simulink model "DC_Motor_Cascade_vs_Single_PI"  (R2021a)
settings: Solver=FixedStepAuto  StartTime=0.0  StopTime=3  FixedStep=1e-4  RelTol=1e-3
values from neighbouring files (symbols this model uses):
  B = 0.002    [motor_params.m]
  J = 0.05    [motor_params.m]
  Ke = 1.5    [motor_params.m]
  Kt = 1.5    [motor_params.m]
  L = 0.02    [motor_params.m]
  R = 2.5    [motor_params.m]
  V_nom = 240    [motor_params.m]
libraries: pid_lib x3, simulink x2
settings Model: SimulationMode=accelerator  Creator=DELL  LastModifiedBy=DELL

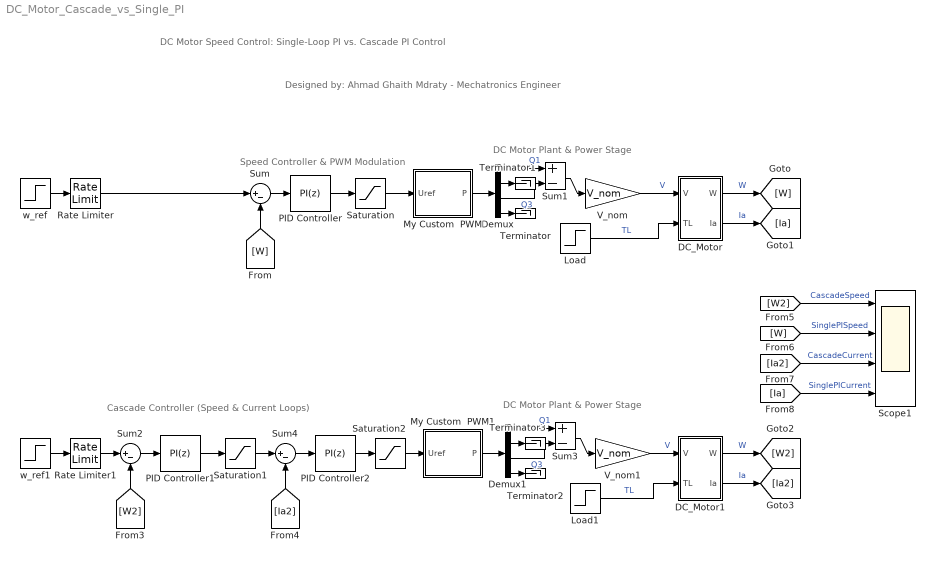
== system DC_Motor_Cascade_vs_Single_PI ==
  note: DC Motor Speed Control: Single-Loop PI vs. Cascade PI Control
  note: DC Motor Plant & Power Stage
  note: Cascade Controller (Speed & Current Loops)
  note: DC Motor Plant & Power Stage
  note: Speed Controller & PWM Modulation
  note: Designed by: Ahmad Ghaith Mdraty - Mechatronics Engineer
  DC_Motor : Subsystem
  DC_Motor1 : Subsystem
  Demux : Demux
  Demux1 : Demux
  Load : Step  Time=2  Before=1  After=20  SampleTime=0
  Load1 : Step  Time=2  Before=1  After=20  SampleTime=0
  My Custom  PWM : Subsystem  mask{PWM_Mode=Unipolar}
      mask prompts: PWM_Mode "Select PWM Modulation:"
      mask TypeOptions PWM_Mode: Bipolar | Unipolar
  My Custom  PWM1 : Subsystem  mask{PWM_Mode=Unipolar}
      mask prompts: PWM_Mode "Select PWM Modulation:"
      mask TypeOptions PWM_Mode: Bipolar | Unipolar
  PID Controller : pid_lib/PID Controller  Controller=PI  Form=Parallel  TimeDomain=Discrete-time  UseExternalTs=off  SampleTime=-1  IntegratorMethod=Forward Euler  FilterMethod=Forward Euler  ControllerParametersSource=internal  P=0.05  I=2  D=0  UseFilter=on  N=100  TunerSelectOption=Transfer Function Based (PID Tuner App)  InitialConditionSource=internal  InitialConditionForIntegrator=0  InitialConditionForFilter=0  DifferentiatorICPrevScaledInput=0  ExternalReset=none  TrackingMode=off  Kt=1  LimitOutput=off  SatLimitsSource=internal  UpperSaturationLimit=inf  LowerSaturationLimit=-inf  LinearizeAsGain=on  AntiWindupMode=none  Kb=1  POutMin=[]  POutMax=[]  IOutMin=[]  IOutMax=[]  DOutMin=[]  DOutMax=[]  NOutMin=[]  NOutMax=[]  SumOutMin=[]  SumOutMax=[]  SaturationOutMin=[]  SaturationOutMax=[]  PParamMin=[]  PParamMax=[]  IParamMin=[]  IParamMax=[]  DParamMin=[]  DParamMax=[]  NParamMin=[]  NParamMax=[]  KbParamMin=[]  KbParamMax=[]  KtParamMin=[]  KtParamMax=[]  KbOutMin=[]  KbOutMax=[]  KtOutMin=[]  KtOutMax=[]  IntegratorOutMin=[]  IntegratorOutMax=[]  FilterOutMin=[]  FilterOutMax=[]  SumI1OutMin=[]  SumI1OutMax=[]  SumI2OutMin=[]  SumI2OutMax=[]  SumI3OutMin=[]  SumI3OutMax=[]  SumI4OutMin=[]  SumI4OutMax=[]  SumDOutMin=[]  SumDOutMax=[]  DifferentiatorOutMin=[]  DifferentiatorOutMax=[]  FilterDiffOutCoefMin=[]  FilterDiffOutCoefMax=[]  ReciprocalOutMin=[]  ReciprocalOutMax=[]  SumDenOutMin=[]  SumDenOutMax=[]  SumNumOutMin=[]  SumNumOutMax=[]  DivideOutMin=[]  DivideOutMax=[]  UdiffTsProdOutMin=[]  UdiffTsProdOutMax=[]  NTsProdOutMin=[]  NTsProdOutMax=[]  UintegralTsProdOutMin=[]  UintegralTsProdOutMax=[]  UngainTsProdOutMin=[]  UngainTsProdOutMax=[]  IntegratorContinuousStateAttributes=''  IntegratorStateMustResolveToSignalObject=off  IntegratorRTWStateStorageClass=Auto  FilterContinuousStateAttributes=''  FilterStateMustResolveToSignalObject=off  FilterRTWStateStorageClass=Auto  ParallelPVariant=InternalParameters  IdealPVariant=Disabled  IVariant=InternalParameters  DVariant=Disabled  IntegratorVariant=Discrete  SatVariant=Disabled  AWVariant=Passthrough  PCopyVariant=Disabled  TRVariant=Disabled  FdbkBlocksVariant=Forward  IdealPFdbkVariant=Disabled  SatFdbkVariant=Disabled  DerivativeFilterVariant=Disabled  NVariant=Disabled  NCopyVariant=Disabled_SignalSpec  FilterICVariant=Disabled  IntegratorICVariant=InternalICs  ExternalResetVariant=Disabled  TRSumVariant=Passthrough  SumFdbkVariant=Disabled  SumVariant=Sum_PI  TsampFilterVariant=InternalTs  TsampNgainVariant=Passthrough  TsampIntegralVariant=Passthrough  ExternalSaturationOutDataTypeStr=Inherit: Same as second input
  PID Controller1 : pid_lib/PID Controller  Controller=PI  Form=Parallel  TimeDomain=Discrete-time  UseExternalTs=off  SampleTime=-1  IntegratorMethod=Forward Euler  FilterMethod=Forward Euler  ControllerParametersSource=internal  P=8  I=40  D=0  UseFilter=on  N=100  TunerSelectOption=Transfer Function Based (PID Tuner App)  InitialConditionSource=internal  InitialConditionForIntegrator=0  InitialConditionForFilter=0  DifferentiatorICPrevScaledInput=0  ExternalReset=none  TrackingMode=off  Kt=1  LimitOutput=off  SatLimitsSource=internal  UpperSaturationLimit=inf  LowerSaturationLimit=-inf  LinearizeAsGain=on  AntiWindupMode=none  Kb=1  POutMin=[]  POutMax=[]  IOutMin=[]  IOutMax=[]  DOutMin=[]  DOutMax=[]  NOutMin=[]  NOutMax=[]  SumOutMin=[]  SumOutMax=[]  SaturationOutMin=[]  SaturationOutMax=[]  PParamMin=[]  PParamMax=[]  IParamMin=[]  IParamMax=[]  DParamMin=[]  DParamMax=[]  NParamMin=[]  NParamMax=[]  KbParamMin=[]  KbParamMax=[]  KtParamMin=[]  KtParamMax=[]  KbOutMin=[]  KbOutMax=[]  KtOutMin=[]  KtOutMax=[]  IntegratorOutMin=[]  IntegratorOutMax=[]  FilterOutMin=[]  FilterOutMax=[]  SumI1OutMin=[]  SumI1OutMax=[]  SumI2OutMin=[]  SumI2OutMax=[]  SumI3OutMin=[]  SumI3OutMax=[]  SumI4OutMin=[]  SumI4OutMax=[]  SumDOutMin=[]  SumDOutMax=[]  DifferentiatorOutMin=[]  DifferentiatorOutMax=[]  FilterDiffOutCoefMin=[]  FilterDiffOutCoefMax=[]  ReciprocalOutMin=[]  ReciprocalOutMax=[]  SumDenOutMin=[]  SumDenOutMax=[]  SumNumOutMin=[]  SumNumOutMax=[]  DivideOutMin=[]  DivideOutMax=[]  UdiffTsProdOutMin=[]  UdiffTsProdOutMax=[]  NTsProdOutMin=[]  NTsProdOutMax=[]  UintegralTsProdOutMin=[]  UintegralTsProdOutMax=[]  UngainTsProdOutMin=[]  UngainTsProdOutMax=[]  IntegratorContinuousStateAttributes=''  IntegratorStateMustResolveToSignalObject=off  IntegratorRTWStateStorageClass=Auto  FilterContinuousStateAttributes=''  FilterStateMustResolveToSignalObject=off  FilterRTWStateStorageClass=Auto  ParallelPVariant=InternalParameters  IdealPVariant=Disabled  IVariant=InternalParameters  DVariant=Disabled  IntegratorVariant=Discrete  SatVariant=Disabled  AWVariant=Passthrough  PCopyVariant=Disabled  TRVariant=Disabled  FdbkBlocksVariant=Forward  IdealPFdbkVariant=Disabled  SatFdbkVariant=Disabled  DerivativeFilterVariant=Disabled  NVariant=Disabled  NCopyVariant=Disabled_SignalSpec  FilterICVariant=Disabled  IntegratorICVariant=InternalICs  ExternalResetVariant=Disabled  TRSumVariant=Passthrough  SumFdbkVariant=Disabled  SumVariant=Sum_PI  TsampFilterVariant=InternalTs  TsampNgainVariant=Passthrough  TsampIntegralVariant=Passthrough  ExternalSaturationOutDataTypeStr=Inherit: Same as second input
  PID Controller2 : pid_lib/PID Controller  Controller=PI  Form=Parallel  TimeDomain=Discrete-time  UseExternalTs=off  SampleTime=-1  IntegratorMethod=Forward Euler  FilterMethod=Forward Euler  ControllerParametersSource=internal  P=0.1  I=15  D=0  UseFilter=on  N=100  TunerSelectOption=Transfer Function Based (PID Tuner App)  InitialConditionSource=internal  InitialConditionForIntegrator=0  InitialConditionForFilter=0  DifferentiatorICPrevScaledInput=0  ExternalReset=none  TrackingMode=off  Kt=1  LimitOutput=off  SatLimitsSource=internal  UpperSaturationLimit=inf  LowerSaturationLimit=-inf  LinearizeAsGain=on  AntiWindupMode=none  Kb=1  POutMin=[]  POutMax=[]  IOutMin=[]  IOutMax=[]  DOutMin=[]  DOutMax=[]  NOutMin=[]  NOutMax=[]  SumOutMin=[]  SumOutMax=[]  SaturationOutMin=[]  SaturationOutMax=[]  PParamMin=[]  PParamMax=[]  IParamMin=[]  IParamMax=[]  DParamMin=[]  DParamMax=[]  NParamMin=[]  NParamMax=[]  KbParamMin=[]  KbParamMax=[]  KtParamMin=[]  KtParamMax=[]  KbOutMin=[]  KbOutMax=[]  KtOutMin=[]  KtOutMax=[]  IntegratorOutMin=[]  IntegratorOutMax=[]  FilterOutMin=[]  FilterOutMax=[]  SumI1OutMin=[]  SumI1OutMax=[]  SumI2OutMin=[]  SumI2OutMax=[]  SumI3OutMin=[]  SumI3OutMax=[]  SumI4OutMin=[]  SumI4OutMax=[]  SumDOutMin=[]  SumDOutMax=[]  DifferentiatorOutMin=[]  DifferentiatorOutMax=[]  FilterDiffOutCoefMin=[]  FilterDiffOutCoefMax=[]  ReciprocalOutMin=[]  ReciprocalOutMax=[]  SumDenOutMin=[]  SumDenOutMax=[]  SumNumOutMin=[]  SumNumOutMax=[]  DivideOutMin=[]  DivideOutMax=[]  UdiffTsProdOutMin=[]  UdiffTsProdOutMax=[]  NTsProdOutMin=[]  NTsProdOutMax=[]  UintegralTsProdOutMin=[]  UintegralTsProdOutMax=[]  UngainTsProdOutMin=[]  UngainTsProdOutMax=[]  IntegratorContinuousStateAttributes=''  IntegratorStateMustResolveToSignalObject=off  IntegratorRTWStateStorageClass=Auto  FilterContinuousStateAttributes=''  FilterStateMustResolveToSignalObject=off  FilterRTWStateStorageClass=Auto  ParallelPVariant=InternalParameters  IdealPVariant=Disabled  IVariant=InternalParameters  DVariant=Disabled  IntegratorVariant=Discrete  SatVariant=Disabled  AWVariant=Passthrough  PCopyVariant=Disabled  TRVariant=Disabled  FdbkBlocksVariant=Forward  IdealPFdbkVariant=Disabled  SatFdbkVariant=Disabled  DerivativeFilterVariant=Disabled  NVariant=Disabled  NCopyVariant=Disabled_SignalSpec  FilterICVariant=Disabled  IntegratorICVariant=InternalICs  ExternalResetVariant=Disabled  TRSumVariant=Passthrough  SumFdbkVariant=Disabled  SumVariant=Sum_PI  TsampFilterVariant=InternalTs  TsampNgainVariant=Passthrough  TsampIntegralVariant=Passthrough  ExternalSaturationOutDataTypeStr=Inherit: Same as second input
  Rate Limiter : RateLimiter  RisingSlewLimit=50  FallingSlewLimit=-50  SampleTimeMode=inherited
  Rate Limiter1 : RateLimiter  RisingSlewLimit=50  FallingSlewLimit=-50  SampleTimeMode=inherited
  Saturation : Saturate  UpperLimit=1  LowerLimit=-1
  Saturation1 : Saturate  UpperLimit=15  LowerLimit=-15
  Saturation2 : Saturate  UpperLimit=1  LowerLimit=-1
  Scope1 : Scope  NumInputPorts=4
  Sum : Sum  Inputs=|+-
  Sum1 : Sum  Inputs=+-  OutDataTypeStr=double
  Sum2 : Sum  Inputs=|+-
  Sum3 : Sum  Inputs=+-  OutDataTypeStr=double
  Sum4 : Sum  Inputs=|+-
  Terminator{,1..3} (4 alike) : Terminator
  V_nom : Gain  Gain=V_nom
  V_nom1 : Gain  Gain=V_nom
  w_ref : Step  Time=0.5  After=50  SampleTime=0
  w_ref1 : Step  Time=0.5  After=50  SampleTime=0
  wires:
  DC_Motor/1(W) -> [W]  "W"
  DC_Motor/2(Ia) -> [Ia]  "Ia"
  [W] -> Sum/2
  V_nom/1 -> DC_Motor/1(V)  "V"
  Load/1 -> DC_Motor/2(TL)  "TL"
  Sum/1 -> PID Controller/1
  Saturation/1 -> My Custom  PWM/1(Uref)
  Demux/2 -> Terminator1/1
  Demux/3 -> Sum1/2  "Q3"
  PID Controller/1 -> Saturation/1
  My Custom  PWM/1(P) -> Demux/1
  w_ref/1 -> Rate Limiter/1
  Rate Limiter/1 -> Sum/1
  Demux/4 -> Terminator/1
  Demux/1 -> Sum1/1  "Q1"
  Sum1/1 -> V_nom/1
  Demux1/4 -> Terminator2/1
  Rate Limiter1/1 -> Sum2/1
  My Custom  PWM1/1(P) -> Demux1/1
  w_ref1/1 -> Rate Limiter1/1
  Demux1/2 -> Terminator3/1
  PID Controller1/1 -> Saturation1/1
  Demux1/3 -> Sum3/2  "Q3"
  DC_Motor1/1(W) -> [W2]  "W"
  Sum2/1 -> PID Controller1/1
  Sum3/1 -> V_nom1/1
  DC_Motor1/2(Ia) -> [Ia2]  "Ia"
  Load1/1 -> DC_Motor1/2(TL)  "TL"
  V_nom1/1 -> DC_Motor1/1(V)  "V"
  [W2] -> Sum2/2
  Demux1/1 -> Sum3/1  "Q1"
  Saturation1/1 -> Sum4/1
  [Ia2] -> Sum4/2
  Sum4/1 -> PID Controller2/1
  PID Controller2/1 -> Saturation2/1
  Saturation2/1 -> My Custom  PWM1/1(Uref)
  [W2] -> Scope1/1  "CascadeSpeed"
  [W] -> Scope1/2  "SinglePISpeed"
  [Ia2] -> Scope1/3  "CascadeCurrent"
  [Ia] -> Scope1/4  "SinglePICurrent"

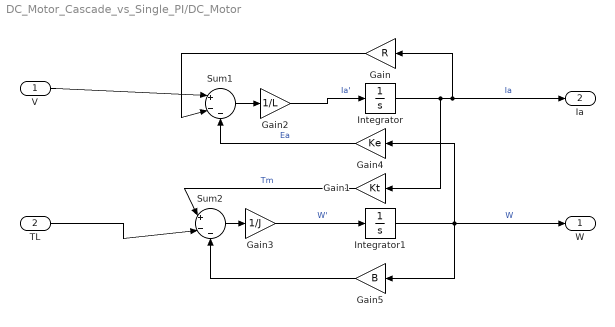
== system DC_Motor_Cascade_vs_Single_PI/DC_Motor ==
  V : Inport
  TL : Inport  Port=2
  Gain : Gain  Gain=R
  Gain1 : Gain  Gain=Kt
  Gain2 : Gain  Gain=1/L
  Gain3 : Gain  Gain=1/J
  Gain4 : Gain  Gain=Ke
  Gain5 : Gain  Gain=B
  Integrator : Integrator
  Integrator1 : Integrator
  Sum1 : Sum  Inputs=|+--
  Sum2 : Sum  Inputs=|+--
  W : Outport
  Ia : Outport  Port=2
  wires:
  TL/1 -> Sum2/2
  Integrator1/1 -> W/1, Gain5/1, Gain4/1  "W"
  Sum1/1 -> Gain2/1
  Gain/1 -> Sum1/2
  V/1 -> Sum1/1
  Gain5/1 -> Sum2/3
  Gain1/1 -> Sum2/1  "Tm"
  Gain4/1 -> Sum1/3  "Ea"
  Sum2/1 -> Gain3/1
  Integrator/1 -> Gain1/1, Ia/1, Gain/1  "Ia"
  Gain3/1 -> Integrator1/1  "W'"
  Gain2/1 -> Integrator/1  "Ia'"

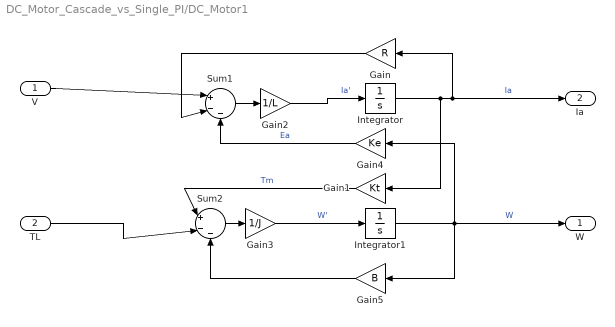
== system DC_Motor_Cascade_vs_Single_PI/DC_Motor1 ==
  V : Inport
  TL : Inport  Port=2
  Gain : Gain  Gain=R
  Gain1 : Gain  Gain=Kt
  Gain2 : Gain  Gain=1/L
  Gain3 : Gain  Gain=1/J
  Gain4 : Gain  Gain=Ke
  Gain5 : Gain  Gain=B
  Integrator : Integrator
  Integrator1 : Integrator
  Sum1 : Sum  Inputs=|+--
  Sum2 : Sum  Inputs=|+--
  W : Outport
  Ia : Outport  Port=2
  wires:
  TL/1 -> Sum2/2
  Integrator1/1 -> W/1, Gain5/1, Gain4/1  "W"
  Sum1/1 -> Gain2/1
  Gain/1 -> Sum1/2
  V/1 -> Sum1/1
  Gain5/1 -> Sum2/3
  Gain1/1 -> Sum2/1  "Tm"
  Gain4/1 -> Sum1/3  "Ea"
  Sum2/1 -> Gain3/1
  Integrator/1 -> Gain1/1, Ia/1, Gain/1  "Ia"
  Gain3/1 -> Integrator1/1  "W'"
  Gain2/1 -> Integrator/1  "Ia'"

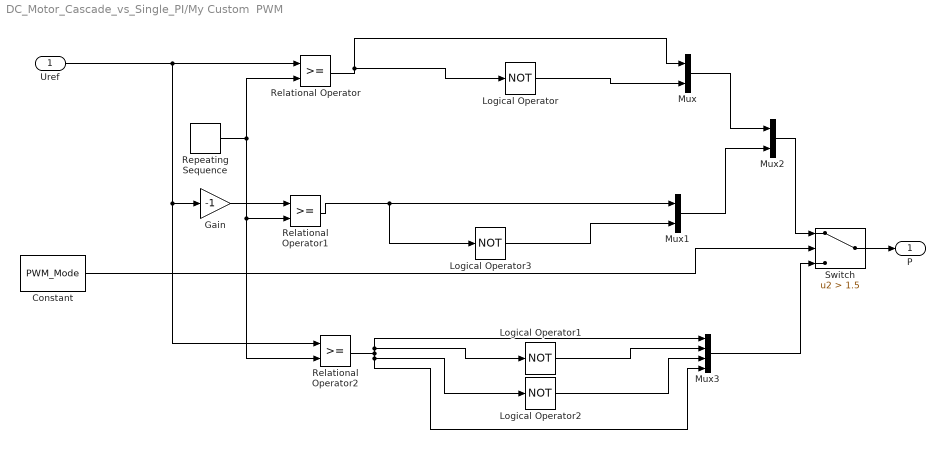
== system DC_Motor_Cascade_vs_Single_PI/My Custom  PWM ==
  Uref : Inport
  Constant : Constant  Value=PWM_Mode
  Gain : Gain  Gain=-1
  Logical Operator{,1..3} (4 alike) : Logic  Operator=NOT  Inputs=1  AllPortsSameDT=off  OutDataTypeStr=boolean
  Mux : Mux  Inputs=2
  Mux1 : Mux  Inputs=2
  Mux2 : Mux  Inputs=2
  Mux3 : Mux
  Relational Operator : RelationalOperator  OutDataTypeStr=boolean  RndMeth=Simplest
  Relational Operator1 : RelationalOperator  OutDataTypeStr=boolean  RndMeth=Simplest
  Relational Operator2 : RelationalOperator  OutDataTypeStr=boolean  RndMeth=Simplest
  Repeating Sequence : simulink/Sources/Repeating Sequence  rep_seq_t="[0  1/(2*5000)  1/5000]"  rep_seq_y="[-1  1  -1]"
  Switch : Switch  Criteria=u2 > Threshold  Threshold=1.5
  P : Outport
  wires:
  Logical Operator/1 -> Mux/2
  Relational Operator/1 -> Logical Operator/1, Mux/1
  Gain/1 -> Relational Operator1/1
  Uref/1 -> Relational Operator/1, Relational Operator2/1, Gain/1
  Relational Operator1/1 -> Logical Operator3/1, Mux1/1
  Logical Operator3/1 -> Mux1/2
  Mux/1 -> Mux2/1
  Mux1/1 -> Mux2/2
  Logical Operator2/1 -> Mux3/3
  Logical Operator1/1 -> Mux3/2
  Repeating Sequence/1 -> Relational Operator1/2, Relational Operator2/2, Relational Operator/2
  Relational Operator2/1 -> Logical Operator1/1, Mux3/1, Logical Operator2/1, Mux3/4
  Mux3/1 -> Switch/3
  Switch/1 -> P/1
  Mux2/1 -> Switch/1
  Constant/1 -> Switch/2

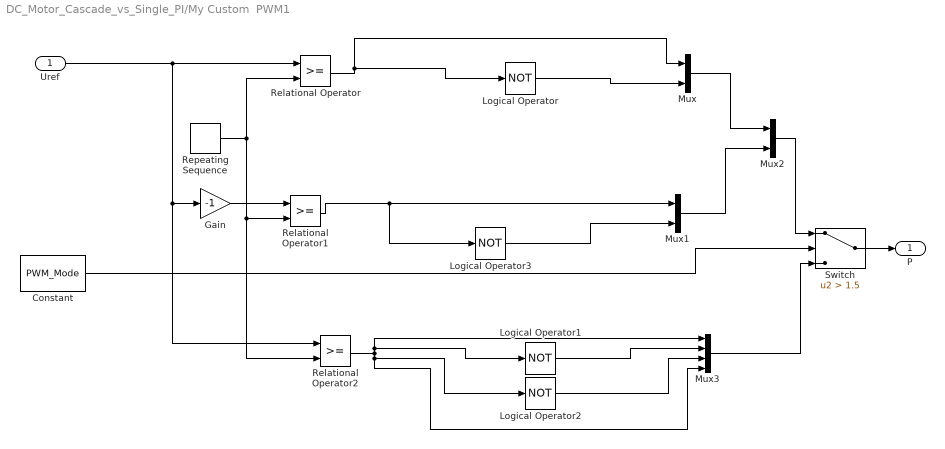
== system DC_Motor_Cascade_vs_Single_PI/My Custom  PWM1 ==
  Uref : Inport
  Constant : Constant  Value=PWM_Mode
  Gain : Gain  Gain=-1
  Logical Operator{,1..3} (4 alike) : Logic  Operator=NOT  Inputs=1  AllPortsSameDT=off  OutDataTypeStr=boolean
  Mux : Mux  Inputs=2
  Mux1 : Mux  Inputs=2
  Mux2 : Mux  Inputs=2
  Mux3 : Mux
  Relational Operator : RelationalOperator  OutDataTypeStr=boolean  RndMeth=Simplest
  Relational Operator1 : RelationalOperator  OutDataTypeStr=boolean  RndMeth=Simplest
  Relational Operator2 : RelationalOperator  OutDataTypeStr=boolean  RndMeth=Simplest
  Repeating Sequence : simulink/Sources/Repeating Sequence  rep_seq_t="[0  1/(2*5000)  1/5000]"  rep_seq_y="[-1  1  -1]"
  Switch : Switch  Criteria=u2 > Threshold  Threshold=1.5
  P : Outport
  wires:
  Logical Operator/1 -> Mux/2
  Relational Operator/1 -> Logical Operator/1, Mux/1
  Gain/1 -> Relational Operator1/1
  Uref/1 -> Relational Operator/1, Relational Operator2/1, Gain/1
  Relational Operator1/1 -> Logical Operator3/1, Mux1/1
  Logical Operator3/1 -> Mux1/2
  Mux/1 -> Mux2/1
  Mux1/1 -> Mux2/2
  Logical Operator2/1 -> Mux3/3
  Logical Operator1/1 -> Mux3/2
  Repeating Sequence/1 -> Relational Operator1/2, Relational Operator2/2, Relational Operator/2
  Relational Operator2/1 -> Logical Operator1/1, Mux3/1, Logical Operator2/1, Mux3/4
  Mux3/1 -> Switch/3
  Switch/1 -> P/1
  Mux2/1 -> Switch/1
  Constant/1 -> Switch/2
